simulink model "hw3_cmg"  (R2022b)
settings: Solver=ode45  StartTime=0.0  StopTime=20.0  RelTol=1e-8  AbsTol=1e-8
undefined symbols (not defined in the file): cmg, orbit, sat, wheel
libraries: matrix_library x1
settings Model: Creator=gagandeepthapar  LastModifiedBy=gagandeepthapar

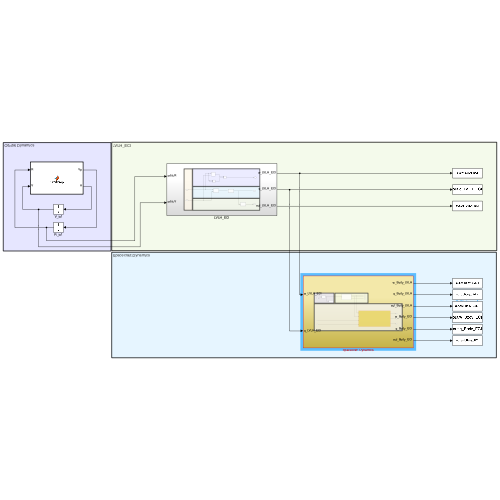
[thumbnail: Simulink's stored preview of the top-level diagram]
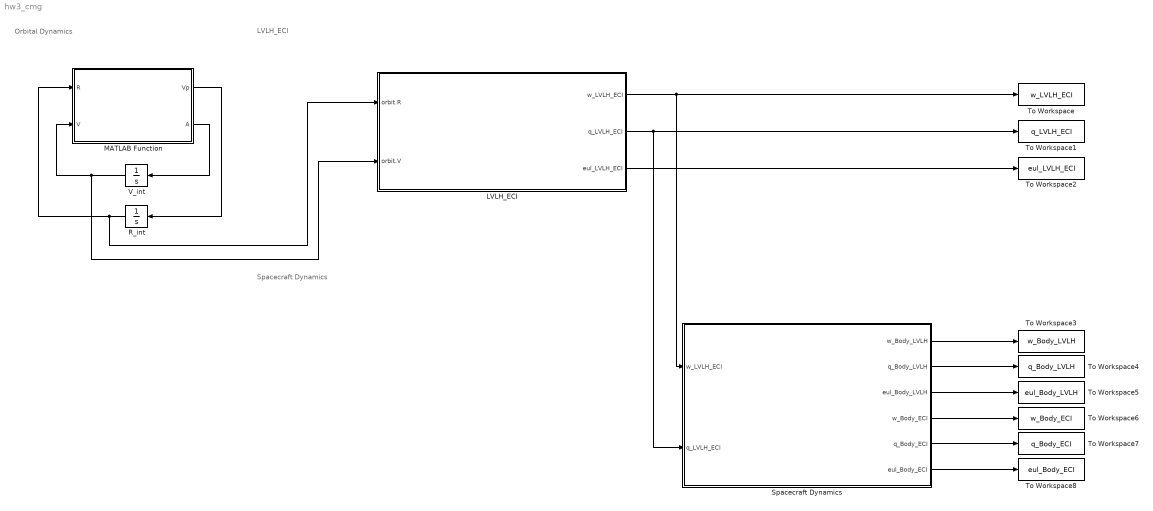
== system hw3_cmg ==
  note: Spacecraft Dynamics
  note: LVLH_ECI
  note: Orbital Dynamics
  LVLH_ECI : Subsystem
  MATLAB Function : MATLAB Function  TreatAsAtomicUnit=on
  R_int : Integrator  InitialCondition=orbit.R0
  Spacecraft Dynamics : Subsystem
  To Workspace : ToWorkspace  VariableName=w_LVLH_ECI  SampleTime=-1
      settings: Save2DSignal=2-D array (concatenate along first dimension)
  To Workspace1 : ToWorkspace  VariableName=q_LVLH_ECI  SampleTime=-1
      settings: Save2DSignal=2-D array (concatenate along first dimension)
  To Workspace2 : ToWorkspace  VariableName=eul_LVLH_ECI  SampleTime=-1
      settings: Save2DSignal=2-D array (concatenate along first dimension)
  To Workspace3 : ToWorkspace  VariableName=w_Body_LVLH  SampleTime=-1
      settings: Save2DSignal=2-D array (concatenate along first dimension)
  To Workspace4 : ToWorkspace  VariableName=q_Body_LVLH  SampleTime=-1
      settings: Save2DSignal=2-D array (concatenate along first dimension)
  To Workspace5 : ToWorkspace  VariableName=eul_Body_LVLH  SampleTime=-1
      settings: Save2DSignal=2-D array (concatenate along first dimension)
  To Workspace6 : ToWorkspace  VariableName=w_Body_ECI  SampleTime=-1
      settings: Save2DSignal=2-D array (concatenate along first dimension)
  To Workspace7 : ToWorkspace  VariableName=q_Body_ECI  SampleTime=-1
      settings: Save2DSignal=2-D array (concatenate along first dimension)
  To Workspace8 : ToWorkspace  VariableName=eul_Body_ECI  SampleTime=-1
      settings: Save2DSignal=2-D array (concatenate along first dimension)
  V_int : Integrator  InitialCondition=orbit.V0
  wires:
  V_int/1 -> MATLAB Function/2(V), LVLH_ECI/2(orbit.V)
  MATLAB Function/2(A) -> V_int/1
  MATLAB Function/1(Vp) -> R_int/1
  R_int/1 -> MATLAB Function/1(R), LVLH_ECI/1(orbit.R)
  LVLH_ECI/3(eul_LVLH_ECI) -> To Workspace2/1
  LVLH_ECI/1(w_LVLH_ECI) -> To Workspace/1, Spacecraft Dynamics/1(w_LVLH_ECI)
  Spacecraft Dynamics/1(w_Body_LVLH) -> To Workspace3/1
  Spacecraft Dynamics/2(q_Body_LVLH) -> To Workspace4/1
  Spacecraft Dynamics/3(eul_Body_LVLH) -> To Workspace5/1
  Spacecraft Dynamics/5(q_Body_ECI) -> To Workspace7/1
  LVLH_ECI/2(q_LVLH_ECI) -> To Workspace1/1, Spacecraft Dynamics/2(q_LVLH_ECI)
  Spacecraft Dynamics/6(eul_Body_ECI) -> To Workspace8/1
  Spacecraft Dynamics/4(w_Body_ECI) -> To Workspace6/1

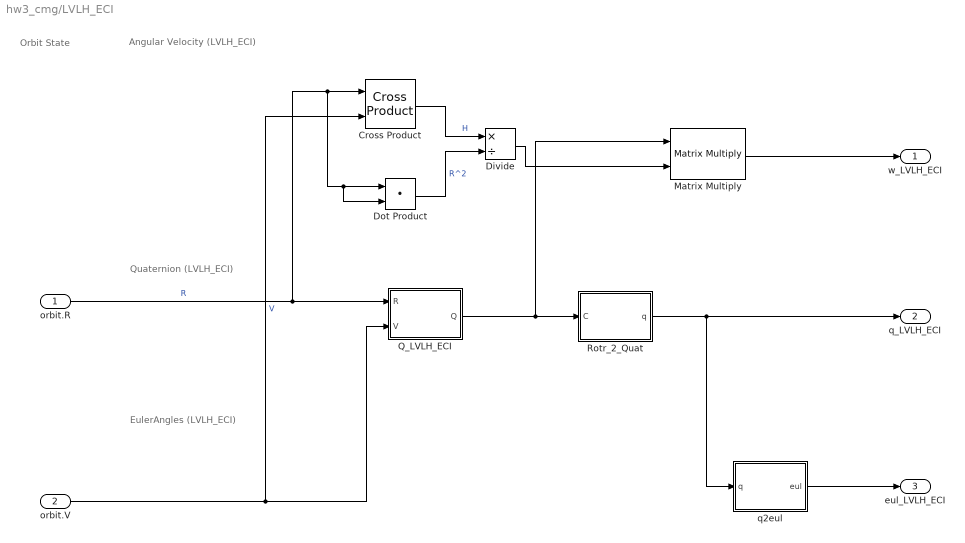
== system hw3_cmg/LVLH_ECI ==
  note: EulerAngles (LVLH_ECI)
  note: Orbit State
  note: Quaternion (LVLH_ECI)
  note: Angular Velocity (LVLH_ECI)
  orbit.R : Inport
  orbit.V : Inport  Port=2
  Cross Product : matrix_library/Cross Product
  Divide : Product  Inputs=*/
  Dot Product : DotProduct  OutDataTypeStr=Inherit: Inherit via internal rule
  Matrix Multiply : Product  Multiplication=Matrix(*)
  Q_LVLH_ECI : MATLAB Function  TreatAsAtomicUnit=on
  Rotr_2_Quat : MATLAB Function  TreatAsAtomicUnit=on
  q2eul : MATLAB Function  TreatAsAtomicUnit=on
  w_LVLH_ECI : Outport
  q_LVLH_ECI : Outport  Port=2
  eul_LVLH_ECI : Outport  Port=3
  wires:
  orbit.R/1 -> Q_LVLH_ECI/1(R), Cross Product/1, Dot Product/1, Dot Product/2  "R"
  orbit.V/1 -> Cross Product/2, Q_LVLH_ECI/2(V)  "V"
  Q_LVLH_ECI/1(Q) -> Matrix Multiply/1, Rotr_2_Quat/1(C)
  Rotr_2_Quat/1(q) -> q2eul/1(q), q_LVLH_ECI/1
  q2eul/1(eul) -> eul_LVLH_ECI/1
  Cross Product/1 -> Divide/1  "H"
  Dot Product/1 -> Divide/2  "R^2"
  Divide/1 -> Matrix Multiply/2
  Matrix Multiply/1 -> w_LVLH_ECI/1

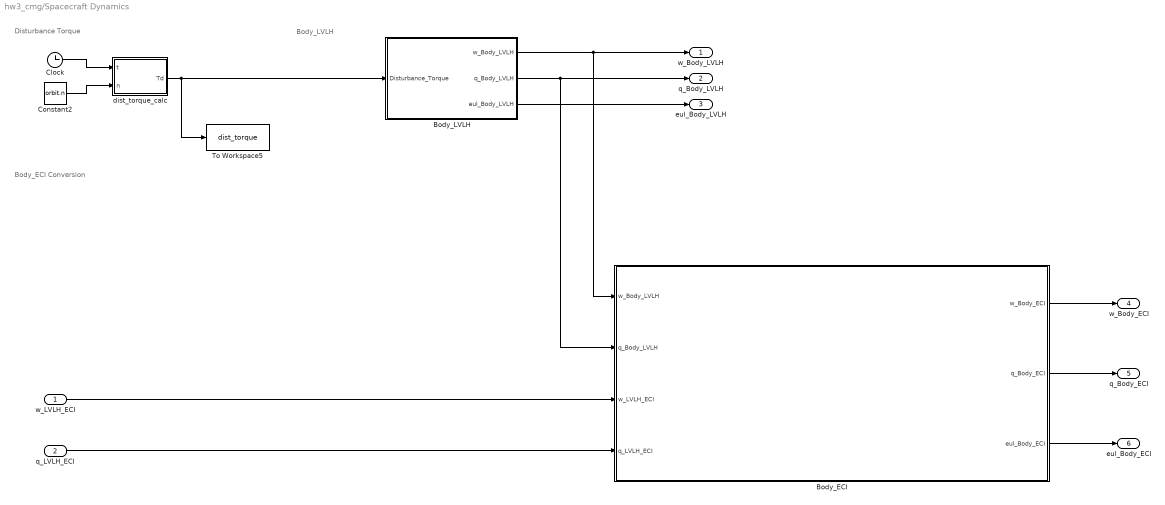
== system hw3_cmg/Spacecraft Dynamics ==
  note: Body_ECI Conversion
  note: Body_LVLH
  note: Disturbance Torque
  w_LVLH_ECI : Inport
  q_LVLH_ECI : Inport  Port=2
  Body_ECI : Subsystem
  Body_LVLH : Subsystem
  Clock : Clock
  Constant2 : Constant  Value=orbit.n
  To Workspace5 : ToWorkspace  VariableName=dist_torque  SampleTime=-1
      settings: Save2DSignal=2-D array (concatenate along first dimension)
  dist_torque_calc : MATLAB Function  TreatAsAtomicUnit=on
  w_Body_LVLH : Outport
  q_Body_LVLH : Outport  Port=2
  eul_Body_LVLH : Outport  Port=3
  w_Body_ECI : Outport  Port=4
  q_Body_ECI : Outport  Port=5
  eul_Body_ECI : Outport  Port=6
  wires:
  Body_LVLH/1(w_Body_LVLH) -> w_Body_LVLH/1, Body_ECI/1(w_Body_LVLH)
  Body_LVLH/2(q_Body_LVLH) -> Body_ECI/2(q_Body_LVLH), q_Body_LVLH/1
  Body_LVLH/3(eul_Body_LVLH) -> eul_Body_LVLH/1
  Body_ECI/2(q_Body_ECI) -> q_Body_ECI/1
  Constant2/1 -> dist_torque_calc/2(n)
  Clock/1 -> dist_torque_calc/1(t)
  q_LVLH_ECI/1 -> Body_ECI/4(q_LVLH_ECI)
  w_LVLH_ECI/1 -> Body_ECI/3(w_LVLH_ECI)
  Body_ECI/1(w_Body_ECI) -> w_Body_ECI/1
  Body_ECI/3(eul_Body_ECI) -> eul_Body_ECI/1
  dist_torque_calc/1(Td) -> Body_LVLH/1(Disturbance_Torque), To Workspace5/1

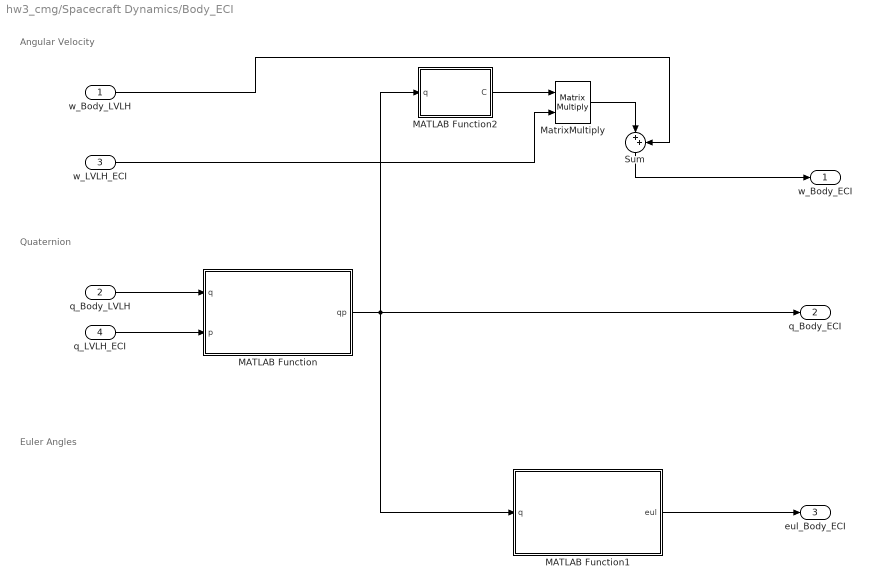
== system hw3_cmg/Spacecraft Dynamics/Body_ECI ==
  note: Quaternion
  note: Euler Angles
  note: Angular Velocity
  w_Body_LVLH : Inport
  q_Body_LVLH : Inport  Port=2
  w_LVLH_ECI : Inport  Port=3
  q_LVLH_ECI : Inport  Port=4
  MATLAB Function : MATLAB Function  TreatAsAtomicUnit=on
  MATLAB Function1 : MATLAB Function  TreatAsAtomicUnit=on
  MATLAB Function2 : MATLAB Function  TreatAsAtomicUnit=on
  MatrixMultiply : Product  Multiplication=Matrix(*)
  Sum : Sum  Inputs=|++
  w_Body_ECI : Outport
  q_Body_ECI : Outport  Port=2
  eul_Body_ECI : Outport  Port=3
  wires:
  q_Body_LVLH/1 -> MATLAB Function/1(q)
  MATLAB Function/1(qp) -> MATLAB Function2/1(q), MATLAB Function1/1(q), q_Body_ECI/1
  q_LVLH_ECI/1 -> MATLAB Function/2(p)
  MATLAB Function1/1(eul) -> eul_Body_ECI/1
  Sum/1 -> w_Body_ECI/1
  MATLAB Function2/1(C) -> MatrixMultiply/1
  w_LVLH_ECI/1 -> MatrixMultiply/2
  MatrixMultiply/1 -> Sum/1
  w_Body_LVLH/1 -> Sum/2

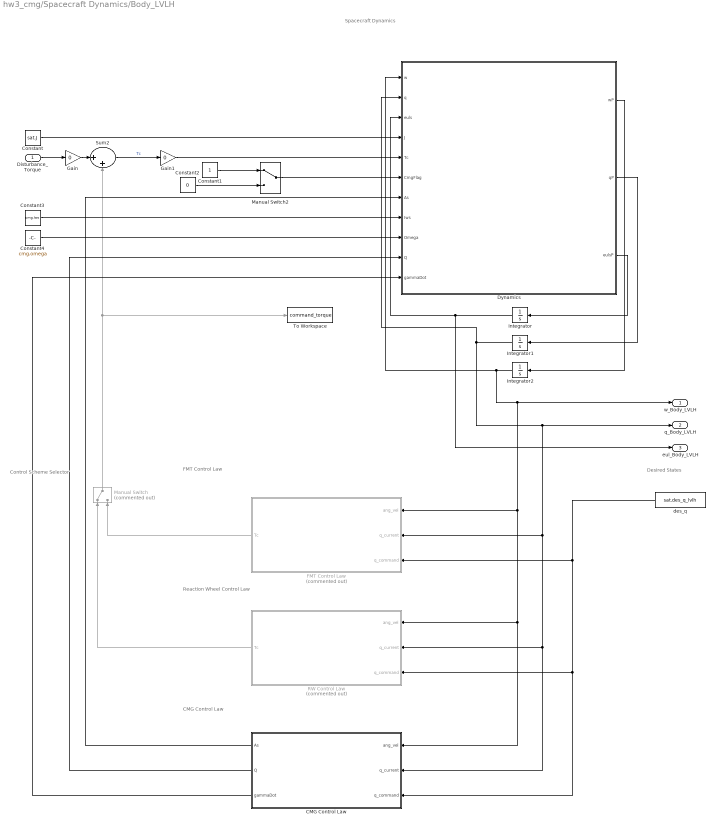
== system hw3_cmg/Spacecraft Dynamics/Body_LVLH ==
  note: Desired States
  note: Control Scheme Selector
  note: Spacecraft Dynamics
  note: FMT Control Law
  note: Reaction Wheel Control Law
  note: CMG Control Law
  Disturbance_Torque : Inport
  CMG Control Law : Subsystem
  Constant : Constant  Value=sat.J
  Constant1 : Constant
  Constant2 : Constant  Value=0
  Constant3 : Constant  Value=cmg.Iws
  Constant4 : Constant  Value=cmg.omega
  Dynamics : MATLAB Function  TreatAsAtomicUnit=on
  FMT Control Law : Subsystem  Commented=on
  Gain : Gain  Gain=0
  Gain1 : Gain  Gain=0
  Integrator : Integrator  InitialCondition=sat.euls0_lvlh
  Integrator1 : Integrator  InitialCondition=[sat.e0_lvlh;sat.n0_lvlh]
  Integrator2 : Integrator  InitialCondition=sat.w0_lvlh
  Manual Switch : ManualSwitch  Commented=on
  Manual Switch2 : ManualSwitch
  RW Control Law : Subsystem  Commented=on
  Sum2 : Sum  Inputs=|++
  To Workspace : ToWorkspace  VariableName=command_torque  SampleTime=-1
      settings: Save2DSignal=2-D array (concatenate along first dimension)
  des_q : Constant  Value=sat.des_q_lvlh
  w_Body_LVLH : Outport
  q_Body_LVLH : Outport  Port=2
  eul_Body_LVLH : Outport  Port=3
  wires:
  Dynamics/3(eulsP) -> Integrator/1
  Dynamics/2(qP) -> Integrator1/1
  Dynamics/1(wP) -> Integrator2/1
  Integrator/1 -> eul_Body_LVLH/1, Dynamics/3(euls)
  Integrator1/1 -> q_Body_LVLH/1, CMG Control Law/2(q_current), RW Control Law/2(q_current), FMT Control Law/2(q_current), Dynamics/2(q)
  Constant/1 -> Dynamics/4(J)
  Integrator2/1 -> w_Body_LVLH/1, CMG Control Law/1(ang_vel), RW Control Law/1(ang_vel), FMT Control Law/1(ang_vel), Dynamics/1(w)
  FMT Control Law/1(Tc) -> Manual Switch/2
  Manual Switch/1 -> To Workspace/1, Sum2/2
  des_q/1 -> CMG Control Law/3(q_command), RW Control Law/3(q_command), FMT Control Law/3(q_command)
  RW Control Law/1(Tc) -> Manual Switch/1
  Gain/1 -> Sum2/1
  Disturbance_Torque/1 -> Gain/1
  Manual Switch2/1 -> Dynamics/6(CmgFlag)
  Constant1/1 -> Manual Switch2/1
  Constant2/1 -> Manual Switch2/2
  CMG Control Law/1(As) -> Dynamics/7(As)
  CMG Control Law/2(Q) -> Dynamics/10(Q)
  CMG Control Law/3(gammaDot) -> Dynamics/11(gammaDot)
  Constant3/1 -> Dynamics/8(Iws)
  Constant4/1 -> Dynamics/9(Omega)
  Sum2/1 -> Gain1/1  "Tc"
  Gain1/1 -> Dynamics/5(Tc)

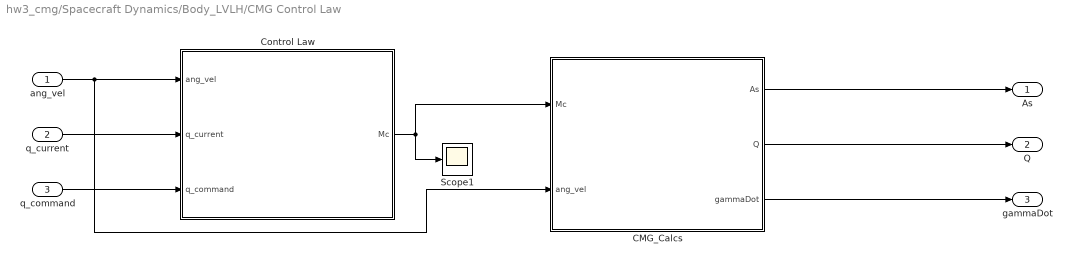
== system hw3_cmg/Spacecraft Dynamics/Body_LVLH/CMG Control Law ==
  ang_vel : Inport
  q_current : Inport  Port=2
  q_command : Inport  Port=3
  CMG_Calcs : Subsystem
  Control Law : Subsystem
  Scope1 : Scope
  As : Outport
  Q : Outport  Port=2
  gammaDot : Outport  Port=3
  wires:
  ang_vel/1 -> CMG_Calcs/2(ang_vel), Control Law/1(ang_vel)
  q_current/1 -> Control Law/2(q_current)
  q_command/1 -> Control Law/3(q_command)
  Control Law/1(Mc) -> Scope1/1, CMG_Calcs/1(Mc)
  CMG_Calcs/1(As) -> As/1
  CMG_Calcs/2(Q) -> Q/1
  CMG_Calcs/3(gammaDot) -> gammaDot/1

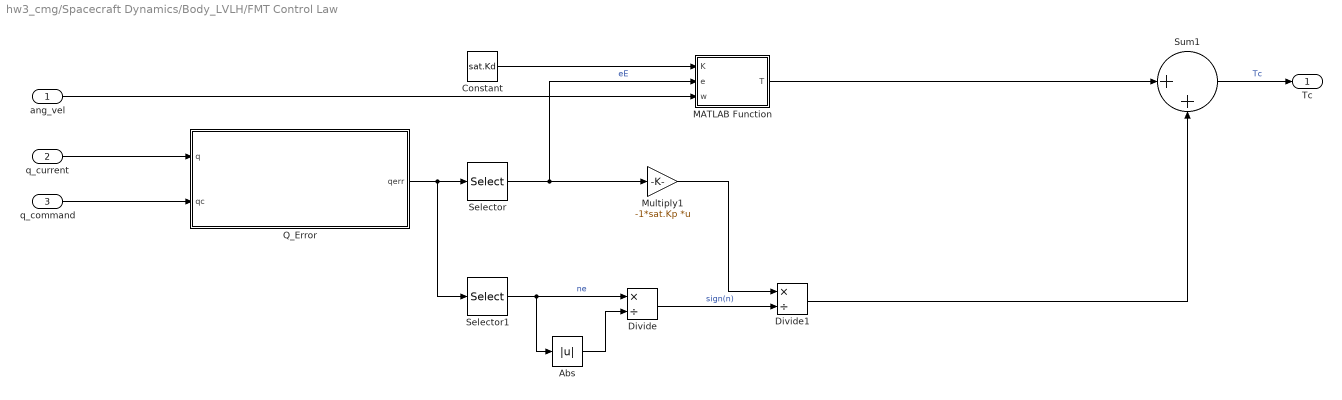
== system hw3_cmg/Spacecraft Dynamics/Body_LVLH/FMT Control Law ==
  ang_vel : Inport
  q_current : Inport  Port=2
  q_command : Inport  Port=3
  Abs : Abs  SaturateOnIntegerOverflow=off
  Constant : Constant  Value=sat.Kd
  Divide : Product  Inputs=*/
  Divide1 : Product  Inputs=*/
  MATLAB Function : MATLAB Function  TreatAsAtomicUnit=on
  Multiply1 : Gain  Gain=-1*sat.Kp  Multiplication=Matrix(K*u)
  Q_Error : MATLAB Function  TreatAsAtomicUnit=on
  Selector : Selector  InputPortWidth=4  IndexOptions=Index vector (dialog)  Indices=[1:3]  OutputSizes=1
  Selector1 : Selector  InputPortWidth=4  IndexOptions=Index vector (dialog)  Indices=[4]  OutputSizes=1
  Sum1 : Sum  Inputs=|++
  Tc : Outport
  wires:
  Sum1/1 -> Tc/1  "Tc"
  q_command/1 -> Q_Error/2(qc)
  Abs/1 -> Divide/2
  Selector/1 -> MATLAB Function/2(e), Multiply1/1  "eE"
  Divide/1 -> Divide1/2  "sign(n)"
  Selector1/1 -> Divide/1, Abs/1  "ne"
  q_current/1 -> Q_Error/1(q)
  Multiply1/1 -> Divide1/1
  Q_Error/1(qerr) -> Selector/1, Selector1/1
  Divide1/1 -> Sum1/2
  MATLAB Function/1(T) -> Sum1/1
  ang_vel/1 -> MATLAB Function/3(w)
  Constant/1 -> MATLAB Function/1(K)

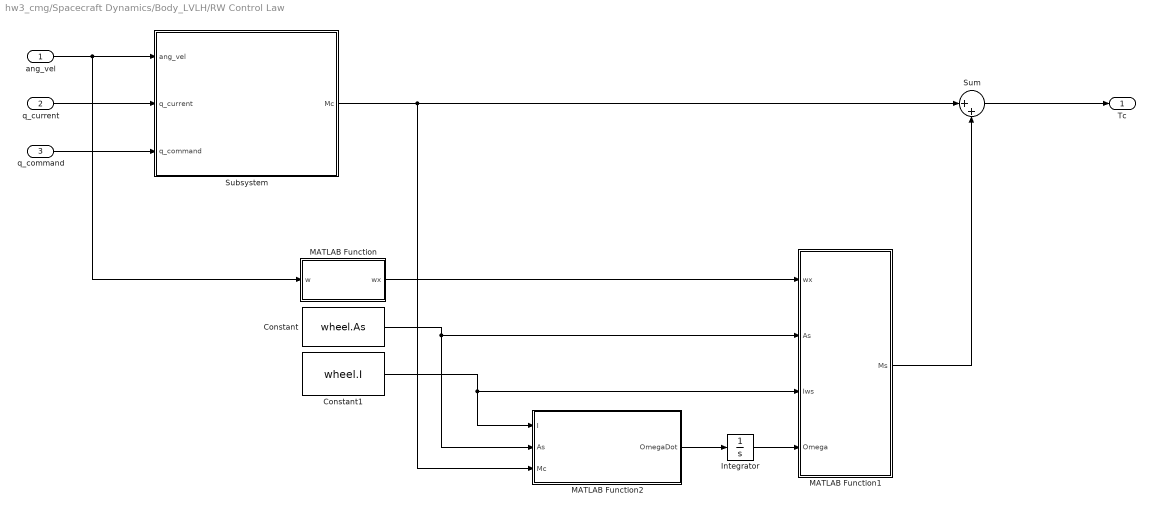
== system hw3_cmg/Spacecraft Dynamics/Body_LVLH/RW Control Law ==
  ang_vel : Inport
  q_current : Inport  Port=2
  q_command : Inport  Port=3
  Constant : Constant  Value=wheel.As  VectorParams1D=off
  Constant1 : Constant  Value=wheel.I
  Integrator : Integrator
  MATLAB Function : MATLAB Function  TreatAsAtomicUnit=on
  MATLAB Function1 : MATLAB Function  TreatAsAtomicUnit=on
  MATLAB Function2 : MATLAB Function  TreatAsAtomicUnit=on
  Subsystem : Subsystem
  Sum : Sum  Inputs=|++
  Tc : Outport
  wires:
  ang_vel/1 -> MATLAB Function/1(w), Subsystem/1(ang_vel)
  q_current/1 -> Subsystem/2(q_current)
  q_command/1 -> Subsystem/3(q_command)
  Sum/1 -> Tc/1
  MATLAB Function1/1(Ms) -> Sum/2
  Subsystem/1(Mc) -> Sum/1, MATLAB Function2/3(Mc)
  Constant/1 -> MATLAB Function2/2(As), MATLAB Function1/2(As)
  MATLAB Function/1(wx) -> MATLAB Function1/1(wx)
  Constant1/1 -> MATLAB Function2/1(I), MATLAB Function1/3(Iws)
  MATLAB Function2/1(OmegaDot) -> Integrator/1
  Integrator/1 -> MATLAB Function1/4(Omega)

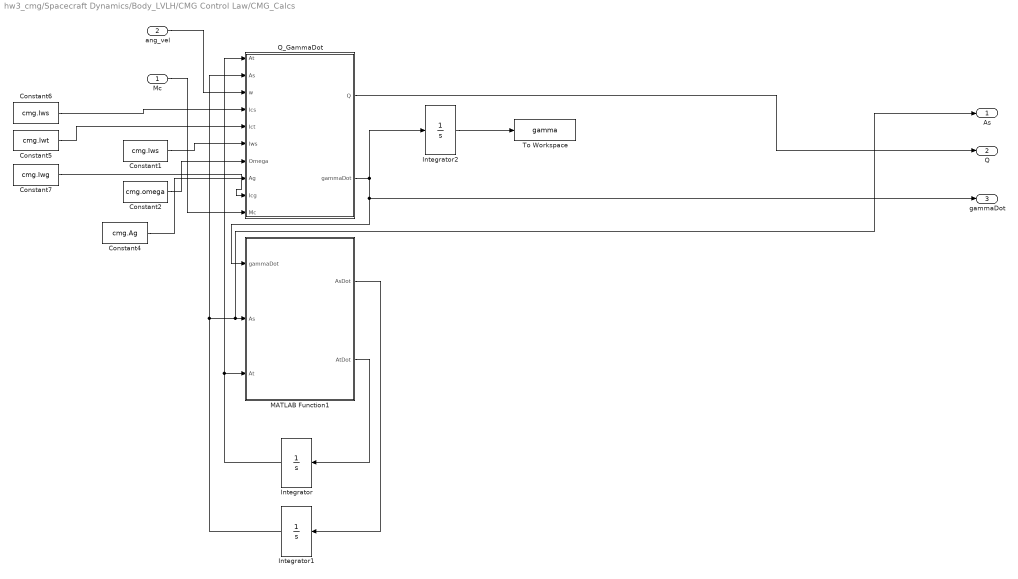
== system hw3_cmg/Spacecraft Dynamics/Body_LVLH/CMG Control Law/CMG_Calcs ==
  Mc : Inport
  ang_vel : Inport  Port=2
  Constant1 : Constant  Value=cmg.Iws
  Constant2 : Constant  Value=cmg.omega
  Constant4 : Constant  Value=cmg.Ag
  Constant5 : Constant  Value=cmg.Iwt
  Constant6 : Constant  Value=cmg.Iws
  Constant7 : Constant  Value=cmg.Iwg
  Integrator : Integrator  InitialCondition=cmg.At
  Integrator1 : Integrator  InitialCondition=cmg.As
  Integrator2 : Integrator  InitialCondition=cmg.gamma
  MATLAB Function1 : MATLAB Function  TreatAsAtomicUnit=on
  Q_GammaDot : MATLAB Function  TreatAsAtomicUnit=on
  To Workspace : ToWorkspace  VariableName=gamma  SampleTime=-1
      settings: Save2DSignal=2-D array (concatenate along first dimension)
  As : Outport
  Q : Outport  Port=2
  gammaDot : Outport  Port=3
  wires:
  Constant1/1 -> Q_GammaDot/6(Iws)
  Constant2/1 -> Q_GammaDot/7(Omega)
  MATLAB Function1/2(AtDot) -> Integrator/1
  Integrator/1 -> MATLAB Function1/3(At), Q_GammaDot/1(At)
  MATLAB Function1/1(AsDot) -> Integrator1/1
  Integrator1/1 -> Q_GammaDot/2(As), As/1, MATLAB Function1/2(As)
  Q_GammaDot/2(gammaDot) -> Integrator2/1, MATLAB Function1/1(gammaDot), gammaDot/1
  Integrator2/1 -> To Workspace/1
  ang_vel/1 -> Q_GammaDot/3(w)
  Constant4/1 -> Q_GammaDot/8(Ag)
  Constant5/1 -> Q_GammaDot/5(Ict)
  Constant6/1 -> Q_GammaDot/4(Ics)
  Constant7/1 -> Q_GammaDot/9(Icg)
  Mc/1 -> Q_GammaDot/10(Mc)
  Q_GammaDot/1(Q) -> Q/1

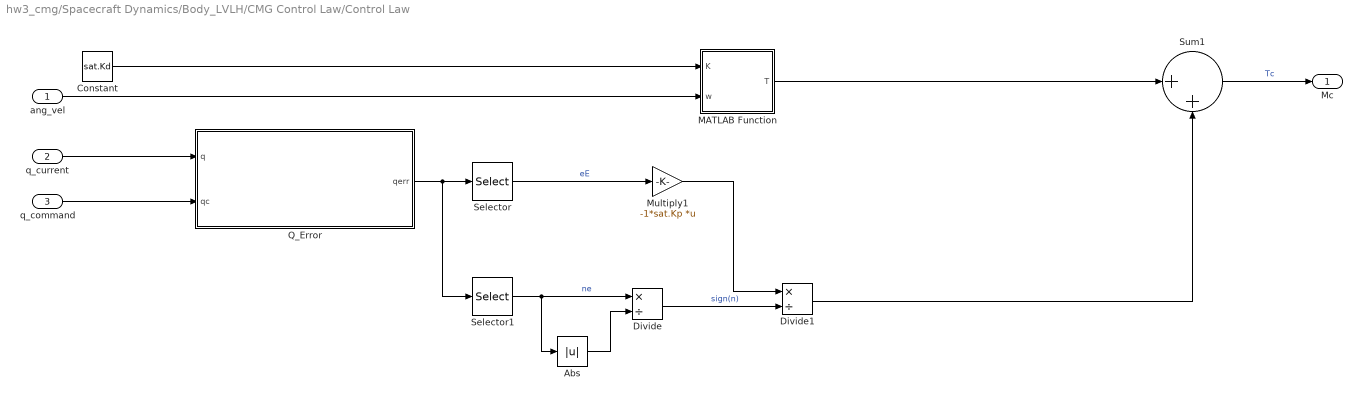
== system hw3_cmg/Spacecraft Dynamics/Body_LVLH/CMG Control Law/Control Law ==
  ang_vel : Inport
  q_current : Inport  Port=2
  q_command : Inport  Port=3
  Abs : Abs  SaturateOnIntegerOverflow=off
  Constant : Constant  Value=sat.Kd
  Divide : Product  Inputs=*/
  Divide1 : Product  Inputs=*/
  MATLAB Function : MATLAB Function  TreatAsAtomicUnit=on
  Multiply1 : Gain  Gain=-1*sat.Kp  Multiplication=Matrix(K*u)
  Q_Error : MATLAB Function  TreatAsAtomicUnit=on
  Selector : Selector  InputPortWidth=4  IndexOptions=Index vector (dialog)  Indices=[1:3]  OutputSizes=1
  Selector1 : Selector  InputPortWidth=4  IndexOptions=Index vector (dialog)  Indices=[4]  OutputSizes=1
  Sum1 : Sum  Inputs=|++
  Mc : Outport
  wires:
  Q_Error/1(qerr) -> Selector/1, Selector1/1
  Sum1/1 -> Mc/1  "Tc"
  Multiply1/1 -> Divide1/1
  Divide/1 -> Divide1/2  "sign(n)"
  Abs/1 -> Divide/2
  Selector/1 -> Multiply1/1  "eE"
  ang_vel/1 -> MATLAB Function/2(w)
  MATLAB Function/1(T) -> Sum1/1
  q_command/1 -> Q_Error/2(qc)
  Selector1/1 -> Divide/1, Abs/1  "ne"
  Constant/1 -> MATLAB Function/1(K)
  q_current/1 -> Q_Error/1(q)
  Divide1/1 -> Sum1/2

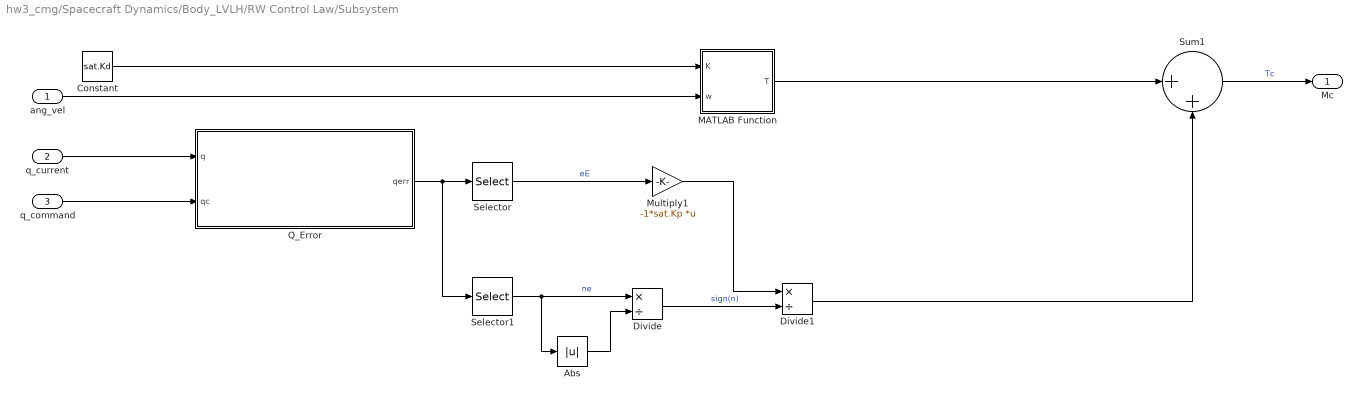
== system hw3_cmg/Spacecraft Dynamics/Body_LVLH/RW Control Law/Subsystem ==
  ang_vel : Inport
  q_current : Inport  Port=2
  q_command : Inport  Port=3
  Abs : Abs  SaturateOnIntegerOverflow=off
  Constant : Constant  Value=sat.Kd
  Divide : Product  Inputs=*/
  Divide1 : Product  Inputs=*/
  MATLAB Function : MATLAB Function  TreatAsAtomicUnit=on
  Multiply1 : Gain  Gain=-1*sat.Kp  Multiplication=Matrix(K*u)
  Q_Error : MATLAB Function  TreatAsAtomicUnit=on
  Selector : Selector  InputPortWidth=4  IndexOptions=Index vector (dialog)  Indices=[1:3]  OutputSizes=1
  Selector1 : Selector  InputPortWidth=4  IndexOptions=Index vector (dialog)  Indices=[4]  OutputSizes=1
  Sum1 : Sum  Inputs=|++
  Mc : Outport
  wires:
  Q_Error/1(qerr) -> Selector/1, Selector1/1
  Sum1/1 -> Mc/1  "Tc"
  Multiply1/1 -> Divide1/1
  Divide/1 -> Divide1/2  "sign(n)"
  Abs/1 -> Divide/2
  Selector/1 -> Multiply1/1  "eE"
  ang_vel/1 -> MATLAB Function/2(w)
  MATLAB Function/1(T) -> Sum1/1
  q_command/1 -> Q_Error/2(qc)
  Selector1/1 -> Divide/1, Abs/1  "ne"
  Constant/1 -> MATLAB Function/1(K)
  q_current/1 -> Q_Error/1(q)
  Divide1/1 -> Sum1/2

== matlab function hw3_cmg/Spacecraft Dynamics/Body_ECI/MATLAB Function2 ==
  data: q input; C output
function C = quat2c(q)

C = quat2rotm([q(4);q(1:3)]');

== matlab function hw3_cmg/Spacecraft Dynamics/Body_LVLH/FMT Control Law/MATLAB Function ==
  data: K input; T output; e input; w input
function T = fcn(K, e, w)

T = -1*K*(1 + e'*e)*w;

== matlab function hw3_cmg/Spacecraft Dynamics/Body_LVLH/RW Control Law/Subsystem/MATLAB Function ==
  data: K input; T output; w input
function T = fcn(K, w)

T = -1*K*w;

== matlab function hw3_cmg/Spacecraft Dynamics/Body_LVLH/RW Control Law/Subsystem/Q_Error ==
  data: q input; qerr output; qc input
function qerr = fcn(q, qc)

%     function wx = skewSymmetric(w)
%         wx = [0, -1*w(3), w(2);
%              w(3), 0, -1*w(1);
%              -1*w(2), w(1), 0];
%     end

    function qp = quatmult(q, p)
    
        function wx = skewSymmetric(w)
            wx = [0, -1*w(3), w(2);
                 w(3), 0, -1*w(1);
                 -1*w(2), w(1), 0];
        end
    
        qn = q(4);
        qe = q(1:3);
    
        pn = p(4);
        pe = p(1:3);
    
        n = pn * qn - pe'*qe;
        e = pn * qe + qn*pe + skewSymmetric(pe)*qe;
    
        qp = [e(1);e(2);e(3);n];
    
    end

qc(1:3) = -1*qc(1:3);
qerr = quatmult(qc, q);

end

== matlab function hw3_cmg/Spacecraft Dynamics/Body_LVLH/RW Control Law/MATLAB Function ==
  data: w input; wx output
function wx = skewSymmetric(w)
        wx = [0, -1*w(3), w(2);
             w(3), 0, -1*w(1);
             -1*w(2), w(1), 0];
end

== matlab function hw3_cmg/Spacecraft Dynamics/Body_LVLH/RW Control Law/MATLAB Function1 ==
  data: wx input; Ms output; As input; Iws input; Omega input
function Ms = Msc_comp(wx, As, Iws, Omega)

Ms = wx*As*Iws*Omega;

end

== matlab function hw3_cmg/Spacecraft Dynamics/Body_LVLH/RW Control Law/MATLAB Function2 ==
  data: I input; As input; Mc input; OmegaDot output
function OmegaDot = OmegaProp(I, As, Mc)

OmegaDot = I\pinv(As)*Mc;

end

== matlab function hw3_cmg/Spacecraft Dynamics/Body_LVLH/CMG Control Law/CMG_Calcs/Q_GammaDot ==
  data: At input size=[3 4]; Q output size=[3 4]; As input size=[3 4]; w input size=[3 1]; Ics input size=[4 4]; Ict input size=[4 4]; gammaDot output size=[4 1]; Iws input size=[4 4]; Omega input size=[4 1]; Ag input size=[3 4]; Icg input size=[4 4]; Mc input size=[3 1]
function [Q, gammaDot] = fcn(At, As, w, Ics, Ict, Iws, Omega, Ag, Icg, Mc)

    function Ad = a_diag(A)
        [x, ~] = size(A);
        X = zeros(x, 3*x);
        for i = 1:x
            X(i, 3*(i-1)+1:3*(i-1)+3) = A(i,:)';
        end
        Ad = X;
    end

    function wx = skewSymmetric(w)
        wx = [0, -1*w(3), w(2);
             w(3), 0, -1*w(1);
             -1*w(2), w(1), 0];
    end

Astd = a_diag(As'); % [As']^d
Attd = a_diag(At'); % [At']^d

a = At*Astd + As*Attd;
b = At * Iws * diag(Omega);
c = skewSymmetric(w)*Ag*Icg;

Q = (a * (kron(eye(4),w)) * (Ics - Ict)) + b + c;

%Q = At*Iws*diag(Omega);

singular = 0.01 * exp(-1*det(Q*Q'));

Qt = inv(Q*Q' + singular*eye(3));

gammaDot = Q'*Qt*Mc;

end

== matlab function hw3_cmg/Spacecraft Dynamics/Body_LVLH/CMG Control Law/CMG_Calcs/MATLAB Function1 ==
  data: gammaDot input; As input; AsDot output; At input; AtDot output
function [AsDot,AtDot] = fcn(gammaDot,As,At)

    AtDot = -1*As*diag(gammaDot);
    AsDot = At * diag(gammaDot);

== matlab function hw3_cmg/Spacecraft Dynamics/Body_LVLH/CMG Control Law/Control Law/MATLAB Function ==
  data: K input; T output; w input
function T = fcn(K, w)

T = -1*K*w;

== matlab function hw3_cmg/Spacecraft Dynamics/Body_LVLH/CMG Control Law/Control Law/Q_Error ==
  data: q input; qerr output; qc input
function qerr = fcn(q, qc)

%     function wx = skewSymmetric(w)
%         wx = [0, -1*w(3), w(2);
%              w(3), 0, -1*w(1);
%              -1*w(2), w(1), 0];
%     end

    function qp = quatmult(q, p)
    
        function wx = skewSymmetric(w)
            wx = [0, -1*w(3), w(2);
                 w(3), 0, -1*w(1);
                 -1*w(2), w(1), 0];
        end
    
        qn = q(4);
        qe = q(1:3);
    
        pn = p(4);
        pe = p(1:3);
    
        n = pn * qn - pe'*qe;
        e = pn * qe + qn*pe + skewSymmetric(pe)*qe;
    
        qp = [e(1);e(2);e(3);n];
    
    end

qc(1:3) = -1*qc(1:3);
qerr = quatmult(qc, q);

end

== matlab function hw3_cmg/LVLH_ECI/Q_LVLH_ECI ==
  data: R input; Q output; V input
function Q = fcn(R,V)


z = -1*R / norm(R);
y = -1 * cross(R,V) / norm(cross(R,V));

x = cross(y,z);

Q = [x,y,z]';

== matlab function hw3_cmg/MATLAB Function ==
  data: R input; Vp output; V input; A output
function [Vp,A] = OrbitProp(R,V)

    mu = 398600;

    rad = norm(R);
    rx = R(1);
    ry = R(2);
    rz = R(3);

    ax = -mu*rx/rad^3;
    ay = -mu*ry/rad^3;
    az = -mu*rz/rad^3;

    Vp = [V(1);V(2);V(3)];
    A = [ax;ay;az];

end

== matlab function hw3_cmg/LVLH_ECI/Rotr_2_Quat ==
  data: C input; q output
function q = fcn(C)

        e = zeros(3,1);
        n = 0.5 * sqrt(1 + trace(C));
        e(1) = 0.25 * (C(2,3) - C(3,2))/n;
        e(2) = 0.25 * (C(3,1) - C(1,3))/n;
        e(3) = 0.25 * (C(1,2) - C(2,1))/n;

        q = [e;n];

== matlab function hw3_cmg/LVLH_ECI/q2eul ==
  data: q input; eul output
function eul = q2eul(q)

    n = q(4);
    e = q(1:3);

    q = [n, e(1), e(2), e(3)];

    phi = atan2(2*(q(1)*q(2) + q(3)*q(4)), 1 - 2*(q(2)^2 + q(3)^2));
    theta = asin(2*(q(1)*q(3) - q(4)*q(2)));
    psi = atan2(2*(q(1)*q(4) + q(2)*q(3)), 1-2*(q(3)^2 + q(4)^2));

    eul = [phi; theta; psi];

== matlab function hw3_cmg/Spacecraft Dynamics/Body_LVLH/Dynamics ==
  data: w input; q input; euls input; wP output; J input; Tc input; CmgFlag input; qP output; eulsP output; As input; Iws input; Omega input; Q input; gammaDot input
function [wP, qP, eulsP] = fcn(w, q, euls, J, Tc, CmgFlag, As, Iws, Omega, Q, gammaDot)
    
    function wx = skewSymmetric(w)
        wx = [0, -1*w(3), w(2);
             w(3), 0, -1*w(1);
             -1*w(2), w(1), 0];
    end

    T = [Tc(1);Tc(2);Tc(3)];

    if CmgFlag == 1

        rhs = skewSymmetric(w)*(J*w + As * Iws * Omega) - Q*gammaDot;
        wP = J\(T - rhs);

    else

        wP = J\(T - skewSymmetric(w)*J*w);

    end

    e = q(1:3);
    n = q(4);
    eP = 0.5*(n*eye(3) + skewSymmetric(e))*w;
    nP = -0.5*e'*w;
    qP = [eP;nP];

    phi = euls(1);
    theta = euls(2);
    psi = euls(3);
    eulsP = 1/(cos(theta)) * [cos(theta), sin(phi)*sin(theta), cos(phi)*sin(theta);
                                0, cos(phi)*cos(theta), -1*sin(phi)*cos(theta);
                                0, sin(phi), cos(phi)] * w;


end

== matlab function hw3_cmg/Spacecraft Dynamics/dist_torque_calc ==
  data: t input; Td output; n input
function Td  = distTorque(t, n)

T = sin(3*n*t)*[0;0.5;0]*10^(-3);
Td = T;
end

== matlab function hw3_cmg/Spacecraft Dynamics/Body_ECI/MATLAB Function ==
  data: q input; qp output; p input
function qp = quatmult(q, p)
    
        function wx = skewSymmetric(w)
            wx = [0, -1*w(3), w(2);
                 w(3), 0, -1*w(1);
                 -1*w(2), w(1), 0];
        end
    
        qn = q(4);
        qe = q(1:3);
    
        pn = p(4);
        pe = p(1:3);
    
        n = pn * qn - pe'*qe;
        e = pn * qe + qn*pe + skewSymmetric(pe)*qe;
    
        qp = [e(1);e(2);e(3);n];

end

== matlab function hw3_cmg/Spacecraft Dynamics/Body_LVLH/FMT Control Law/Q_Error ==
  data: q input; qerr output; qc input
function qerr = fcn(q, qc)

%     function wx = skewSymmetric(w)
%         wx = [0, -1*w(3), w(2);
%              w(3), 0, -1*w(1);
%              -1*w(2), w(1), 0];
%     end

    function qp = quatmult(q, p)
    
        function wx = skewSymmetric(w)
            wx = [0, -1*w(3), w(2);
                 w(3), 0, -1*w(1);
                 -1*w(2), w(1), 0];
        end
    
        qn = q(4);
        qe = q(1:3);
    
        pn = p(4);
        pe = p(1:3);
    
        n = pn * qn - pe'*qe;
        e = pn * qe + qn*pe + skewSymmetric(pe)*qe;
    
        qp = [e(1);e(2);e(3);n];
    
    end

qc(1:3) = -1*qc(1:3);
qerr = quatmult(qc, q);

end

== matlab function hw3_cmg/Spacecraft Dynamics/Body_ECI/MATLAB Function1 ==
  data: q input; eul output
function eul = quat_eul(q)

    n = q(4);
    ex = q(1);
    ey = q(2);
    ez = q(3);

    a = 2*(n*ey - ez*ex);
    if a > 1
        a = 1;
    elseif a < -1
        a = -1;
    end

    phi = atan2(2*(n*ex + ey*ez), 1 - 2*(ex^2 + ey^2));
    theta = asin(a);
    psi = atan2(2*(n*ez + ex*ey), 1 - 2*(ey^2 + ez^2));

    eul = [phi;theta;psi];

end
